simulink model "v3"  (R2019b)
settings: Solver=FixedStepAuto  StartTime=0.0  StopTime=inf  FixedStep=1e-3  RelTol=1e-3  EnableMultiTasking=on
undefined symbols (not defined in the file): D0, D1, D10, D11, D12, D13, D2, D3, D4, D5, D6, D7, D8, D9, PTA0, PTA1, PTA2, PTB23, PTB9, PTC16, PTC17, PTC2, PTC3, PTC4, PTD0, PTD1, PTD2, PTD3
libraries: frdmk64flib x20, nucleoutilitieslib x2
settings Model: ExtModeTrigDuration=5  Creator=zhangg24  LastModifiedBy=Gannonc
settings DataIOCC: ReturnWorkspaceOutputs=off
settings OptimizationCC: PassReuseOutputArgsThreshold=0  MaxStackSize=64
settings DebuggingCC: ParameterTunabilityLossMsg=error  UnderSpecifiedDimensionMsg=warning  ArithmeticOperatorsInVariantConditions=warning
settings HardwareCC: ProdBitPerPointer=32  ProdBitPerSizeT=32  ProdBitPerPtrDiffT=32  ProdLargestAtomicInteger=Long  ProdLargestAtomicFloat=Double  ProdWordSize=32  ProdHWDeviceType=ARM Compatible->ARM Cortex  UseEmbeddedCoderFeatures=off
settings SFSimCC: SimUseLocalCustomCode=off  MATLABDynamicMemAlloc=off  CustomCodeUndefinedFunction=UseInterfaceOnly
settings RTWCC: SystemTargetFile=ert.tlc  HardwareBoard=NXP FRDM-K64F  TLCOptions="-aInlineSetEventsForThisBaseRateFcn=TLC_FALSE -aSuppressMultiTaskScheduler=TLC_FALSE  -aRateBasedStepFcn=0"  TemplateMakefile=ert_default_tmf  GenerateReport=on  RTWUseLocalCustomCode=off  Toolchain=GNU Tools for ARM Embedded Processors  LaunchReport=on
settings CodeAppCC: ForceParamTrailComments=on  OperatorAnnotations=on
settings ERTTargetCC: ERTCustomFileBanners=off  SupportContinuousTime=on  SupportNonInlinedSFcns=on  RemoveResetFunc=off  ModelStepFunctionPrototypeControlCompliant=off

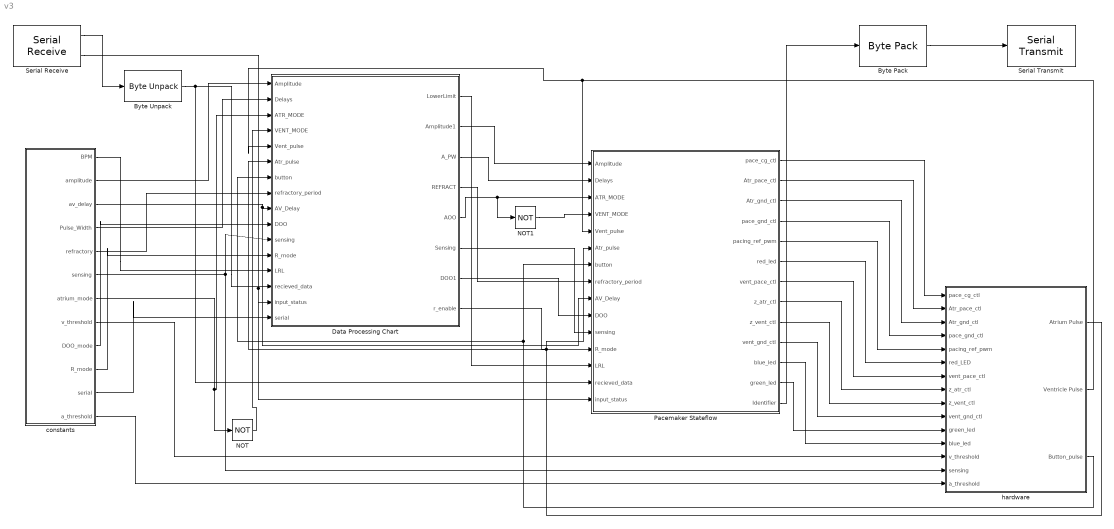
== system v3 ==
  Byte Pack : nucleoutilitieslib/Byte Pack  datatypes={'uint8'}  byteAlign=1  blockPlatform=nucleo
      settings: SourceProductName=Embedded Coder Support Package for ARM Cortex-A Processors  SourceProductBaseCode=ECCORTEXA
  Byte Unpack : nucleoutilitieslib/Byte Unpack  dimensions={[10]}  datatypes={'double'}  byteAlign=1  blockPlatform=nucleo
      settings: SourceProductName=Embedded Coder Support Package for ARM Cortex-A Processors  SourceProductBaseCode=ECCORTEXA
  Data Processing Chart : Stateflow chart  TreatAsAtomicUnit=on
  NOT : Logic  Operator=NOT  IconShape=distinctive  AllPortsSameDT=off  OutDataTypeStr=boolean
  NOT1 : Logic  Operator=NOT  IconShape=distinctive  AllPortsSameDT=off  OutDataTypeStr=boolean
  Pacemaker Stateflow : Stateflow chart  TreatAsAtomicUnit=on
  Serial Receive : frdmk64flib/Serial Receive  SCIModule=0  Baudrate=uint32(9600)  Parity=None  StopBits=1  HardwareFlowControl=None  ByteOrder=LittleEndian  DataType=double  DataLength=10  BlockingMode=off  OutputStatus=on  SampleTime=0.001
      settings: SourceProductName=Simulink Coder Support Package for NXP FRDM-K64F Board
  Serial Transmit : frdmk64flib/Serial Transmit  SCIModule=0  Baudrate=uint32(9600)  Parity=None  StopBits=1  HardwareFlowControl=None  ByteOrder=LittleEndian  BlockingMode=on  OutputStatus=off
      settings: SourceProductName=Simulink Coder Support Package for NXP FRDM-K64F Board
  constants : Subsystem
  hardware : Subsystem
  wires:
  Pacemaker Stateflow/1(pace_cg_ctl) -> hardware/1(pace_cg_ctl)
  Pacemaker Stateflow/2(Atr_pace_ctl) -> hardware/2(Atr_pace_ctl)
  Pacemaker Stateflow/3(Atr_gnd_ctl) -> hardware/3(Atr_gnd_ctl)
  Pacemaker Stateflow/4(pace_gnd_ctl) -> hardware/4(pace_gnd_ctl)
  Pacemaker Stateflow/5(pacing_ref_pwm) -> hardware/5(pacing_ref_pwm)
  Pacemaker Stateflow/7(vent_pace_ctl) -> hardware/7(vent_pace_ctl)
  Pacemaker Stateflow/8(z_atr_ctl) -> hardware/8(z_atr_ctl)
  Pacemaker Stateflow/9(z_vent_ctl) -> hardware/9(z_vent_ctl)
  Pacemaker Stateflow/10(vent_gnd_ctl) -> hardware/10(vent_gnd_ctl)
  Pacemaker Stateflow/6(red_led) -> hardware/6(red_LED)
  Pacemaker Stateflow/11(blue_led) -> hardware/12(blue_led)
  Pacemaker Stateflow/12(green_led) -> hardware/11(green_led)
  hardware/2(Ventricle Pulse) -> Data Processing Chart/5(Vent_pulse), Pacemaker Stateflow/5(Vent_pulse)
  hardware/1(Atrium Pulse) -> Pacemaker Stateflow/6(Atr_pulse), Data Processing Chart/6(Atr_pulse)
  hardware/3(Button_pulse) -> Pacemaker Stateflow/7(button), Data Processing Chart/7(button)
  constants/6(sensing) -> hardware/14(sensing), Data Processing Chart/11(sensing)
  constants/8(v_threshold) -> hardware/13(v_threshold)
  Byte Pack/1 -> Serial Transmit/1
  Pacemaker Stateflow/13(Identifier) -> Byte Pack/1
  Serial Receive/2 -> Data Processing Chart/15(input_status), Pacemaker Stateflow/15(input_status)
  constants/1("BPM ") -> Data Processing Chart/13(LRL)
  constants/2(amplitude) -> Data Processing Chart/1(Amplitude)
  constants/3(av_delay) -> Pacemaker Stateflow/9(AV_Delay), Data Processing Chart/9(AV_Delay)
  constants/4(Pulse_Width) -> Data Processing Chart/2(Delays)
  constants/5(refractory) -> Data Processing Chart/8(refractory_period)
  constants/7(atrium_mode) -> NOT/1, Data Processing Chart/3(ATR_MODE)
  NOT/1 -> Data Processing Chart/4(VENT_MODE)
  constants/9(DOO_mode) -> Data Processing Chart/10(DOO)
  constants/10(R_mode) -> Data Processing Chart/12(R_mode)
  Data Processing Chart/1(LowerLimit) -> Pacemaker Stateflow/13(LRL)
  Data Processing Chart/2(Amplitude1) -> Pacemaker Stateflow/1(Amplitude)
  Data Processing Chart/3(A_PW) -> Pacemaker Stateflow/2(Delays)
  Data Processing Chart/4(REFRACT) -> Pacemaker Stateflow/8(refractory_period)
  Data Processing Chart/7(DOO1) -> Pacemaker Stateflow/10(DOO)
  Data Processing Chart/6(Sensing) -> Pacemaker Stateflow/11(sensing)
  Data Processing Chart/5(AOO) -> NOT1/1, Pacemaker Stateflow/3(ATR_MODE)
  NOT1/1 -> Pacemaker Stateflow/4(VENT_MODE)
  constants/11(serial) -> Data Processing Chart/16(serial)
  Data Processing Chart/8(r_enable) -> Pacemaker Stateflow/12(R_mode)
  constants/12(a_threshold) -> hardware/15(a_threshold)
  Serial Receive/1 -> Byte Unpack/1
  Byte Unpack/1 -> Pacemaker Stateflow/14(recieved_data), Data Processing Chart/14(recieved_data)

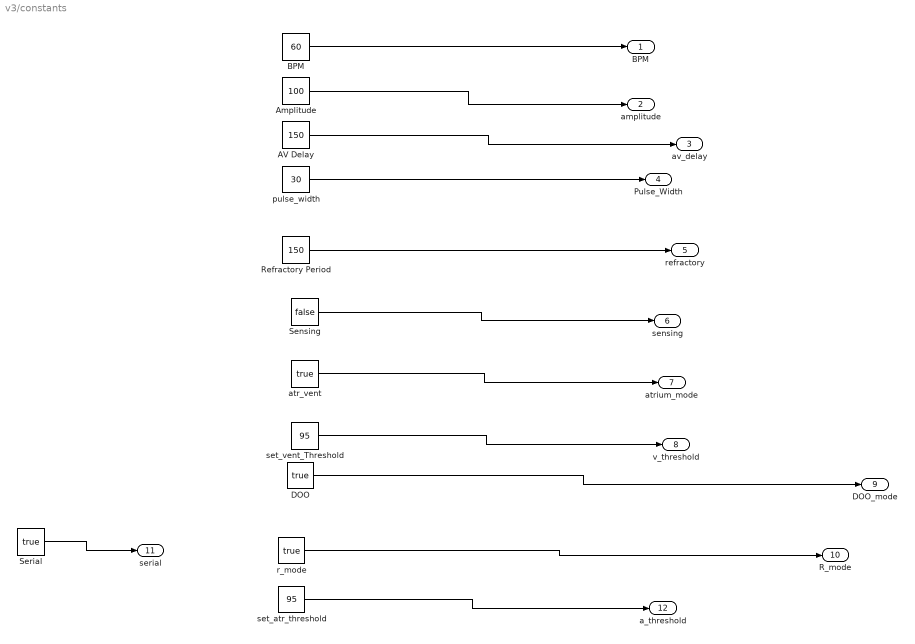
== system v3/constants ==
  AV Delay : Constant  Value=150
  Amplitude : Constant  Value=100  OutDataTypeStr=int16
  BPM : Constant  Value=60  OutDataTypeStr=uint32
  DOO : Constant  Value=true  OutDataTypeStr=boolean
  Refractory Period : Constant  Value=150  OutDataTypeStr=uint32  SampleTime=-1
  Sensing : Constant  Value=false
  Serial : Constant  Value=true
  atr_vent : Constant  Value=true  OutDataTypeStr=boolean
  pulse_width : Constant  Value=30  OutDataTypeStr=uint32
  r_mode : Constant  Value=true  OutDataTypeStr=boolean
  set_atr_threshold : Constant  Value=95
  set_vent_Threshold : Constant  Value=95
  "BPM " : Outport
  amplitude : Outport  Port=2
  av_delay : Outport  Port=3
  Pulse_Width : Outport  Port=4
  refractory : Outport  Port=5
  sensing : Outport  Port=6
  atrium_mode : Outport  Port=7
  v_threshold : Outport  Port=8
  DOO_mode : Outport  Port=9
  R_mode : Outport  Port=10
  serial : Outport  Port=11
  a_threshold : Outport  Port=12
  wires:
  DOO/1 -> DOO_mode/1
  Refractory Period/1 -> refractory/1
  Sensing/1 -> sensing/1
  atr_vent/1 -> atrium_mode/1
  set_vent_Threshold/1 -> v_threshold/1
  AV Delay/1 -> av_delay/1
  BPM/1 -> "BPM "/1
  Amplitude/1 -> amplitude/1
  pulse_width/1 -> Pulse_Width/1
  r_mode/1 -> R_mode/1
  Serial/1 -> serial/1
  set_atr_threshold/1 -> a_threshold/1

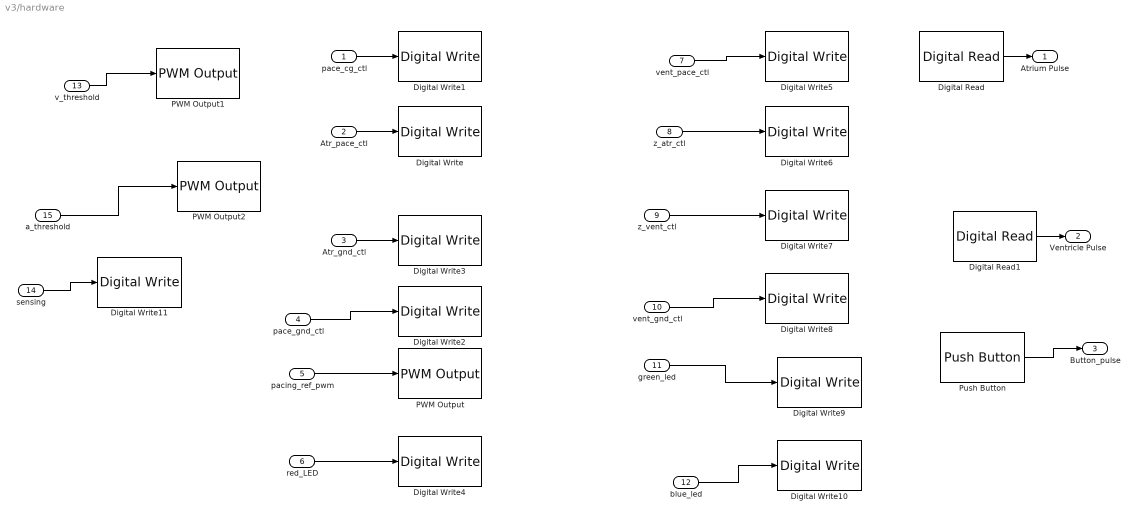
== system v3/hardware ==
  pace_cg_ctl : Inport
  Atr_pace_ctl : Inport  Port=2
  Atr_gnd_ctl : Inport  Port=3
  pace_gnd_ctl : Inport  Port=4
  pacing_ref_pwm : Inport  Port=5
  red_LED : Inport  Port=6
  vent_pace_ctl : Inport  Port=7
  z_atr_ctl : Inport  Port=8
  z_vent_ctl : Inport  Port=9
  vent_gnd_ctl : Inport  Port=10
  green_led : Inport  Port=11
  blue_led : Inport  Port=12
  v_threshold : Inport  Port=13
  sensing : Inport  Port=14
  a_threshold : Inport  Port=15
  Digital Read : frdmk64flib/Digital Read  Whichpin=PTC16 (D0)  SampleTime=-1
      settings: SourceProductName=Simulink Coder Support Package for NXP FRDM-K64F Board
  Digital Read1 : frdmk64flib/Digital Read  Whichpin=PTC17 (D1)  SampleTime=-1
      settings: SourceProductName=Simulink Coder Support Package for NXP FRDM-K64F Board
  Digital Write : frdmk64flib/Digital Write  Whichpin=PTA0 (D8)
      settings: SourceProductName=Simulink Coder Support Package for NXP FRDM-K64F Board
  Digital Write1 : frdmk64flib/Digital Write  Whichpin=PTB9 (D2)
      settings: SourceProductName=Simulink Coder Support Package for NXP FRDM-K64F Board
  Digital Write10 : frdmk64flib/Digital Write  Whichpin=BLUE_LED
      settings: SourceProductName=Simulink Coder Support Package for NXP FRDM-K64F Board
  Digital Write11 : frdmk64flib/Digital Write  Whichpin=PTD1 (D13)
      settings: SourceProductName=Simulink Coder Support Package for NXP FRDM-K64F Board
  Digital Write2 : frdmk64flib/Digital Write  Whichpin=PTD0 (D10)
      settings: SourceProductName=Simulink Coder Support Package for NXP FRDM-K64F Board
  Digital Write3 : frdmk64flib/Digital Write  Whichpin=PTD2 (D11)
      settings: SourceProductName=Simulink Coder Support Package for NXP FRDM-K64F Board
  Digital Write4 : frdmk64flib/Digital Write  Whichpin=RED_LED
      settings: SourceProductName=Simulink Coder Support Package for NXP FRDM-K64F Board
  Digital Write5 : frdmk64flib/Digital Write  Whichpin=PTC4 (D9)
      settings: SourceProductName=Simulink Coder Support Package for NXP FRDM-K64F Board
  Digital Write6 : frdmk64flib/Digital Write  Whichpin=PTB23 (D4)
      settings: SourceProductName=Simulink Coder Support Package for NXP FRDM-K64F Board
  Digital Write7 : frdmk64flib/Digital Write  Whichpin=PTC3 (D7)
      settings: SourceProductName=Simulink Coder Support Package for NXP FRDM-K64F Board
  Digital Write8 : frdmk64flib/Digital Write  Whichpin=PTD3 (D12)
      settings: SourceProductName=Simulink Coder Support Package for NXP FRDM-K64F Board
  Digital Write9 : frdmk64flib/Digital Write  Whichpin=GREEN_LED
      settings: SourceProductName=Simulink Coder Support Package for NXP FRDM-K64F Board
  PWM Output : frdmk64flib/PWM Output  Whichpin=PTA2 (D5)  InitialFrequency=2000  InitialDutyCycle=0
      settings: SourceProductName=Simulink Coder Support Package for NXP FRDM-K64F Board
  PWM Output1 : frdmk64flib/PWM Output  Whichpin=PTA1 (D3)  InitialFrequency=2000  InitialDutyCycle=0
      settings: SourceProductName=Simulink Coder Support Package for NXP FRDM-K64F Board
  PWM Output2 : frdmk64flib/PWM Output  Whichpin=PTC2 (D6)  InitialFrequency=2000  InitialDutyCycle=0
      settings: SourceProductName=Simulink Coder Support Package for NXP FRDM-K64F Board
  Push Button : frdmk64flib/Push Button  Whichswitch=SW2  SampleTime1=-1
      settings: SourceProductName=Simulink Coder Support Package for NXP FRDM-K64F Board
  Atrium Pulse : Outport
  Ventricle Pulse : Outport  Port=2
  Button_pulse : Outport  Port=3
  wires:
  Atr_pace_ctl/1 -> Digital Write/1
  pace_cg_ctl/1 -> Digital Write1/1
  pace_gnd_ctl/1 -> Digital Write2/1
  Atr_gnd_ctl/1 -> Digital Write3/1
  pacing_ref_pwm/1 -> PWM Output/1
  red_LED/1 -> Digital Write4/1
  vent_pace_ctl/1 -> Digital Write5/1
  vent_gnd_ctl/1 -> Digital Write8/1
  z_vent_ctl/1 -> Digital Write7/1
  z_atr_ctl/1 -> Digital Write6/1
  green_led/1 -> Digital Write9/1
  blue_led/1 -> Digital Write10/1
  Digital Read/1 -> Atrium Pulse/1
  Digital Read1/1 -> Ventricle Pulse/1
  v_threshold/1 -> PWM Output1/1
  Push Button/1 -> Button_pulse/1
  sensing/1 -> Digital Write11/1
  a_threshold/1 -> PWM Output2/1

== stateflow chart v3/Data Processing Chart ==
  settings: executeAtInitialization=1
  state INIT
    %Processes incoming data. If data is not recieved from DCM, parameters
    %default to Simulink constants
    entry:
    if recieved_data(1)~=0 && serial
    r_enable=recieved_data(10)
    if recieved_data(6)==1|| recieved_data(6)==3
    AOO=true
    Amplitude1=recieved_data(3)
    A_PW=recieved_data(4)
    REFRACT=recieved_data(5)
    DOO1=false
    else if recieved_data(6)==2|| recieved_data(6)==4
    AOO=false
    Amplitude1=recieved_data(3)
    A_PW=recieved_data(4)
    REFRACT=recieved_data(5)
    DOO1=false
    else
    Amplitude1=recieved_data(3)
    A_PW=recieved_data(4)
    REFRACT=recieved_data(5)
    DOO1=true
    end
    end
    else
    Amplitude1=Amplitude
    LowerLimit=LRL
    A_PW=Delays
    AOO=ATR_MODE
    Sensing=sensing
    DOO1=DOO
    REFRACT=refractory_period
    r_enable=R_mode
    end
  (default) -> INIT
  data: Amplitude input int16; Delays input uint32; ATR_MODE input boolean; VENT_MODE input boolean; Vent_pulse input boolean; Atr_pulse input boolean; button input boolean; refractory_period input uint32; AV_Delay input; DOO input; ATR_STATE local boolean; VENT_STATE local boolean; Initialize local; sensing input; R_mode input; BPM local uint32; data local uint16; pace_cnt_test local double; LRL input; recieved_data input; input_status input; LowerLimit output; Amplitude1 output; A_PW output; REFRACT output uint32; AOO output; Sensing output; DOO1 output; serial input; data1 local; data2 local; r_enable output

== stateflow chart v3/Pacemaker Stateflow ==
  settings: executeAtInitialization=1
  state Sensing_Artificial
    %sensing state following an artificial pace.
    %if no pace is detected, resume artificial pacing
    blue_led=true
    green_led=false
    red_led=false
  state INIT
    %upon initialization, device is in charge mode
    %BPM is converted throughout chart to ms delay
    %Identifier is serially transmitted to identify this device
    entry:
    BPM=LRL
    Atr_pace_ctl=false
    Vent_pace_ctl=false
    pacing_ref_pwm=Amplitude
    pace_cg_ctl=true
    green_led=true
    red_led=false
    blue_led=false
    pace_gnd_ctl=true
    Vent_pace_ctl=false
    z_atr_ctl=false
    z_vent_ctl=false
    Atr_pace_ctl=false
    pacing_ref_pwm=Amplitude
    ATR_STATE=(ATR_MODE||DOO)
    VENT_STATE=(VENT_MODE&&~DOO)
    Atr_gnd_ctl=ATR_STATE
    vent_gnd_ctl=VENT_STATE
    pace_cnt_test=0
    Identifier=42
  state Pace
    %Sends a pace to ATR/VENT
    %chamber is set by ATR_STATE
    %and VENT_STATE
    entry:
    pace_cg_ctl=false
    pace_gnd_ctl=true
    Atr_pace_ctl=ATR_STATE
    Atr_gnd_ctl=false
    z_atr_ctl=false
    z_vent_ctl=false
    vent_gnd_ctl=false
    Vent_pace_ctl=VENT_STATE
    pacing_ref_pwm=Amplitude
    red_led=true
    green_led=false
    blue_led=false
  state Sensing_Natural
    %sensing state following a natural pace.
    %if no pace is detected, resume artificial pacing
    blue_led=true
    green_led=false
    red_led=false
  state Natural_Pace
    %State is entered when natural pace is detected
    %Exits after refratory period to begin pacing/sensing
    red_led=false
    green_led=false
    blue_led=false
  state Charge
    %Charges pacing capacitor
    %if DOO is enabled, it waits based on AV_delay/BPM, and flows to pace
    %if DOO is not enabled, it flows to the sensing states after the refractory period
    entry:
    Atr_pace_ctl=false
    Vent_pace_ctl=false
    pacing_ref_pwm=Amplitude
    pace_cg_ctl=true
    green_led=true
    red_led=false
    blue_led=false
  state Discharge
    %Discharges ground capacitor
    %chamber is set by ATR_STATE
    %and VENT_STATE
    entry:
    pace_gnd_ctl=true
    Vent_pace_ctl=false
    z_atr_ctl=false
    z_vent_ctl=false
    Atr_pace_ctl=false
    pacing_ref_pwm=Amplitude
    Atr_gnd_ctl=ATR_STATE
    vent_gnd_ctl=VENT_STATE
  state Mode_Switch
    %if DOO, flip modes for next pace
    entry:
    ATR_STATE=~ATR_STATE
    VENT_STATE=~VENT_STATE
  Sensing_Artificial -> Pace [order 1] : [after((1000)*60.0/(BPM)-refractory_period, msec)]
  INIT -> Sensing_Artificial [order 1] : [DOO==false&&after(refractory_period-Delays,msec)]
  Charge -> Sensing_Artificial [order 3] : [[DOO==false&&after(refractory_period-Delays,msec)]]
  (default) -> INIT
  Sensing_Artificial -> Natural_Pace [order 2] : [[sensing&&((ATR_MODE ==true && Atr_pulse==true ) || (VENT_MODE ==true && Vent_pulse==true ) || button)]]
  INIT -> Pace [order 2] : [VENT_STATE&&DOO&&after(AV_Delay,msec)]
  INIT -> Pace [order 3] : [[ATR_STATE&&DOO&&after((1000)*60.0/(BPM)-AV_Delay-Delays,msec)]]
  Natural_Pace -> Sensing_Natural : [after(refractory_period,msec)]
  Sensing_Natural -> Natural_Pace [order 1] : [sensing&&((ATR_MODE ==true && Atr_pulse==true ) || (VENT_MODE ==true && Vent_pulse==true ) || button)]
  Charge -> Pace [order 2] : [[VENT_STATE&&DOO&&after(AV_Delay-Delays,msec)]]
  Sensing_Natural -> Pace [order 2] : [[after((1000)*60.0/(BPM)-refractory_period-Delays, msec)]]
  Charge -> Pace [order 1] : [[[ATR_STATE&&DOO&&after((1000)*60.0/(BPM)-AV_Delay-Delays,msec)]]]
  Pace -> Charge [order 1] : [~DOO&&after(Delays, msec)]
  Pace -> Discharge [order 2] : [after(Delays, msec)]
  Mode_Switch -> Charge
  Discharge -> Mode_Switch [order 1] : [DOO]
  Discharge -> Charge [order 2] : [~DOO]
  data: Amplitude input uint8; pace_cg_ctl output boolean; Atr_pace_ctl output boolean; Atr_gnd_ctl output boolean; pace_gnd_ctl output boolean; pacing_ref_pwm output int16; Delays input uint8; red_led output boolean; vent_pace_ctl output boolean; z_atr_ctl output boolean; z_vent_ctl output boolean; vent_gnd_ctl output boolean; ATR_MODE input boolean; VENT_MODE input boolean; blue_led output boolean; green_led output boolean; Vent_pulse input boolean; Atr_pulse input boolean; button input boolean; refractory_period input uint8; AV_Delay input; DOO input; ATR_STATE local boolean; VENT_STATE local boolean; Initialize local; sensing input; R_mode input; BPM local uint8; data local; pace_cnt_test local double; LRL input; Identifier output; recieved_data input; input_status input
